simulink model "Ex5_4"  (R2022b)
settings: Solver=ode4  StartTime=0.0  StopTime=50  FixedStep=0.001  RelTol=1e-3
values from neighbouring files (symbols this model uses):
  par =     [par.mat]
settings Model: Creator=super  LastModifiedBy=15043
settings ModelReferenceCC: EnableRefExpFcnMdlSchedulingChecks=on

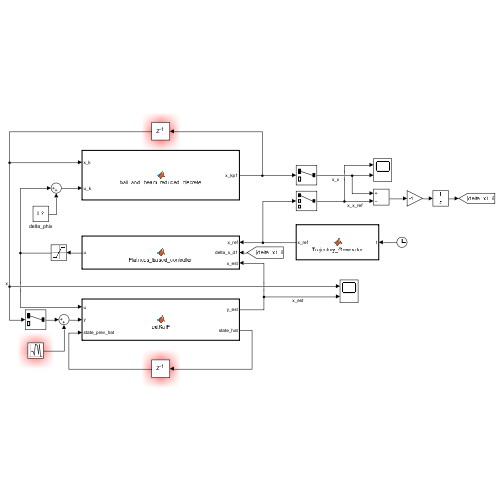
[thumbnail: Simulink's stored preview of the top-level diagram]
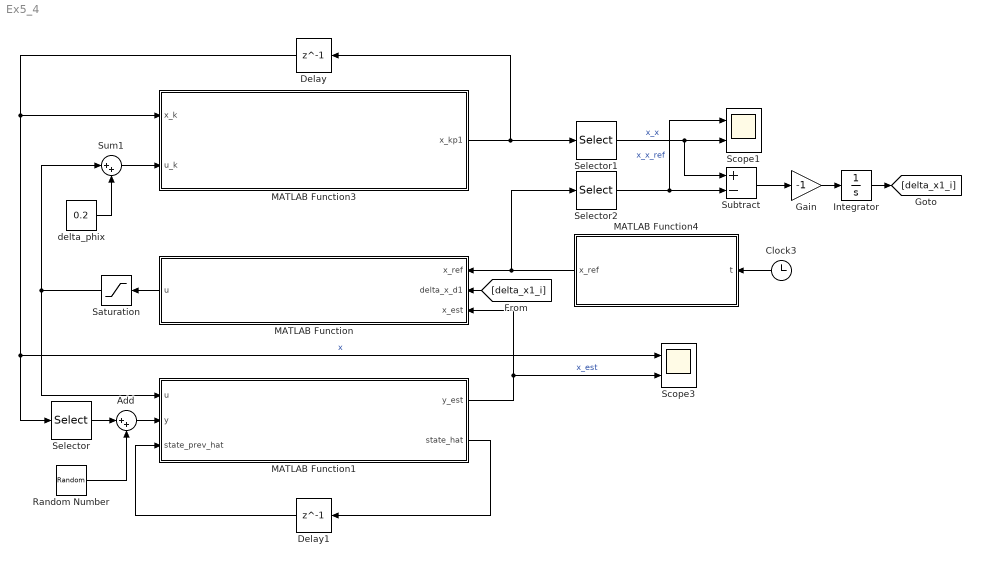
== system Ex5_4 ==
  Add : Sum  Inputs=|++
  Clock3 : Clock
  Delay : Delay  DelayLength=1  InitialCondition=par.ex5_4_x0
  Delay1 : Delay  DelayLength=1  InitialCondition=par.ex5_4_x0_hat  UseCircularBuffer=on
  Gain : Gain  Gain=-1
  Integrator : Integrator
  MATLAB Function : MATLAB Function  TreatAsAtomicUnit=on
  MATLAB Function1 : MATLAB Function  TreatAsAtomicUnit=on
  MATLAB Function3 : MATLAB Function  TreatAsAtomicUnit=on
  MATLAB Function4 : MATLAB Function  TreatAsAtomicUnit=on
  Random Number : RandomNumber  Variance=1e-6  SampleTime=par.timeStep
  Saturation : Saturate  UpperLimit=10  LowerLimit=-10
  Scope1 : Scope  NumInputPorts=2
  Scope3 : Scope  NumInputPorts=2
  Selector : Selector  InputPortWidth=2  IndexOptions=Index vector (dialog)  Indices=[1]  OutputSizes=1
  Selector1 : Selector  InputPortWidth=2  IndexOptions=Index vector (dialog)  Indices=[1]  OutputSizes=1
  Selector2 : Selector  InputPortWidth=3  IndexOptions=Index vector (dialog)  Indices=[1]  OutputSizes=1
  Subtract : Sum  Inputs=+-
  Sum1 : Sum  Inputs=|++
  delta_phix : Constant  Value=0.2
  wires:
  Delay/1 -> Selector/1, Scope3/1, MATLAB Function3/1(x_k)  "x"
  MATLAB Function1/2(state_hat) -> Delay1/1
  Delay1/1 -> MATLAB Function1/3(state_prev_hat)
  MATLAB Function1/1(y_est) -> MATLAB Function/3(x_est), Scope3/2  "x_est"
  MATLAB Function3/1(x_kp1) -> Delay/1, Selector1/1
  Clock3/1 -> MATLAB Function4/1(t)
  MATLAB Function4/1(x_ref) -> MATLAB Function/1(x_ref), Selector2/1
  MATLAB Function/1(u) -> Saturation/1
  Selector1/1 -> Scope1/2, Subtract/1  "x_x"
  Selector2/1 -> Scope1/1, Subtract/2  "x_x_ref"
  Subtract/1 -> Gain/1
  Gain/1 -> Integrator/1
  Integrator/1 -> [delta_x1_i]
  [delta_x1_i] -> MATLAB Function/2(delta_x_d1)
  Selector/1 -> Add/1
  Add/1 -> MATLAB Function1/2(y)
  Random Number/1 -> Add/2
  Saturation/1 -> Sum1/1, MATLAB Function1/1(u)
  delta_phix/1 -> Sum1/2
  Sum1/1 -> MATLAB Function3/2(u_k)

== matlab function Ex5_4/MATLAB Function ==
  data: x_ref input; delta_x_d1 input; x_est input; u output; par parameter
function u = Flatness_based_controller(x_ref, delta_x_d1, x_est, par)
g = par.g;
p1 = par.p1;
p0 = par.p0;

v = x_ref(3) - p1*(x_est(2) - x_ref(2)) - p0*(x_est(1) - x_ref(1)) +50*delta_x_d1;
u = -asin((7*v)/(5*g));
end

== matlab function Ex5_4/MATLAB Function4 ==
  data: t input; x_ref output
function x_ref = Trajectory_Generator(t)

    % Preallocate the reference trajectory and derivatives vector
    x_ref = zeros(3,1);

    % Symbolic expressions as calculated in remark 5.1
    x_ref(1) =  cos((pi*t)/2)/25;
    x_ref(2) = -(pi*sin((pi*t)/2))/50;
    x_ref(3) = -(pi^2*cos((pi*t)/2))/100;

== matlab function Ex5_4/MATLAB Function1 ==
  data: y_est output; u input; state_hat output; y input; state_prev_hat input; par parameter
function [y_est, state_hat] = extKalF(u, y, state_prev_hat, par )
    
    R = par.R;          % Measurement covariance matrix
    Q = par.Q;          % Process covariance matrix

    ts = par.timeStep;  % discretization timestep for the explicit euler

    h = @(x) [x(1)];    % As we only measure the first state
    
    H = [1 0];          % Measurement Jacobian        
    dF = [ 0 1; 0 0];   % State jacobian    
    
    x_hat_prev = state_prev_hat(1:2, :);
    P_prev = reshape( state_prev_hat(3:end), 2,2);
    
    % discretize the nonlinear model
    fd = x_hat_prev + ts*f( x_hat_prev, u, par );
    
    % discretize the jacobian
    F = eye(2) + ts*dF;

    %%%%%% Predict step %%%%%%
    x_hatm = fd;
    Pm = F*P_prev*F' + Q;
    
    %%%%%% Update step %%%%%%
    K = Pm*H'/((H*Pm*H'+ R));         % Kalman gain
    
    x_hat = x_hatm + K*(y-h(x_hatm));   
    P = ( eye(2) - K*H)*Pm ;
         
    state_hat = [x_hat; P(:);];
    y_est = x_hat_prev;
 end


function dx = f( x, u, par )
    
    % system parameters   
    g = par.g;

    % States vector
    x2 = x(2);

    % Preallocate
    dx = zeros(2,1);

    % reduced model
    dx(1) = x2;
    dx(2) = -(5/7)*g*sin(u);
end

== matlab function Ex5_4/MATLAB Function3 ==
  data: x_k input; u_k input; x_kp1 output; par parameter
function x_kp1 = ball_and_beam_reduced_discrete(x_k, u_k, par)
%#codegen
x_kp1 = ball_and_beam_reduced_discrete(x_k, u_k, par);
